simulink model "modelxxx"  (R2023a)
settings: Solver=FixedStepAuto  StartTime=0.0  StopTime=inf  FixedStep=0.001  MaxStep=0.001  RelTol=1e-3
undefined symbols (not defined in the file or in its folder): CR, LF
libraries: instrumentseriallib x2
settings Model: SimulationMode=accelerator  Creator=Adam  LastModifiedBy=Adam
settings SolverCC: AlgebraicLoopSolver=TrustRegion
settings DataIOCC: ExternalInput=ind  SaveOutput=off  SignalLogging=off  DSMLogging=off  SaveTime=off  ReturnWorkspaceOutputs=off  OutputSaveName=out  ReturnWorkspaceOutputsName=sout
settings OptimizationCC: SimCompilerOptimization=on  AccelVerboseBuild=on
settings DebuggingCC: AlgebraicLoopMsg=none  UnconnectedInputMsg=warning  UnconnectedOutputMsg=warning  UnconnectedLineMsg=warning
settings ModelReferenceCC: EnableRefExpFcnMdlSchedulingChecks=on
settings RTWCC: DLArmComputeVersion=19.05

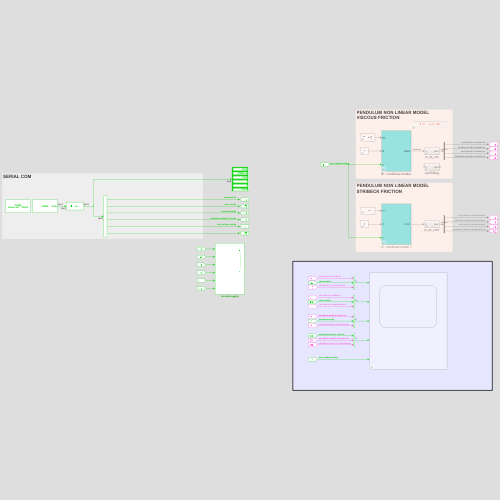
[thumbnail: Simulink's stored preview of the top-level diagram]
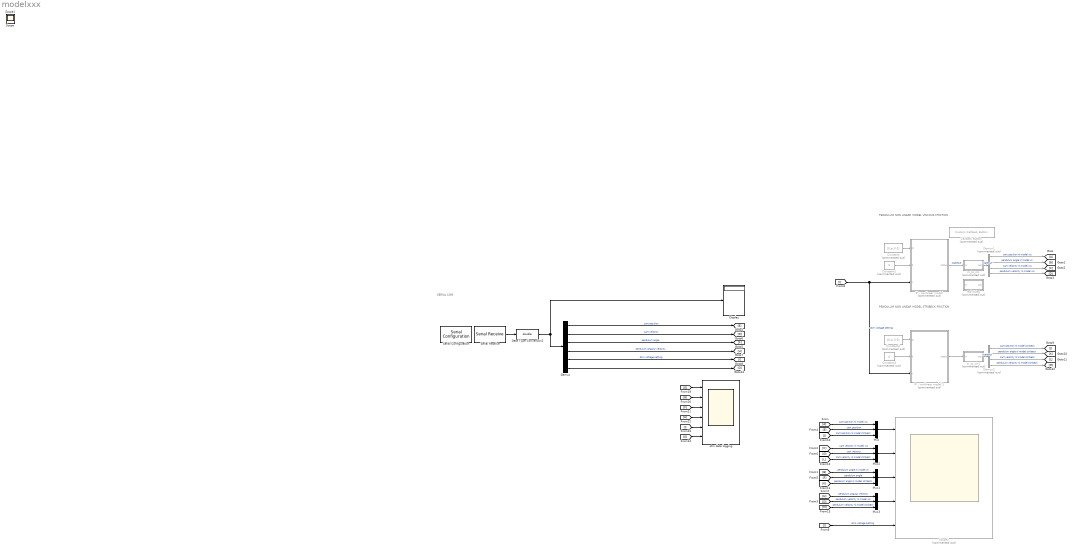
== system modelxxx ==
  note: PENDULUM NON LINEAR MODEL
      | VISCOUS FRICTION
  note: SERIAL COM
  note: PENDULUM NON LINEAR MODEL
      | STRIBECK FRICTION
  Callback Button : CustomCallbackButton  Commented=on  Configuration="{\"components\":[{\"name\":\"BackgroundImageComponent\",\"settings\":{\"image\":{\"size\":[0,0],\"src\":\"default\",\"srcOrientation\":\"Right\"},\"position\":[0,0,1,1]}},{\"name\":\"ButtonStateComponent\",\"settings\":{\"buttonType\":\"momentary\",\"clickFcn\":\"run(\\\"C:\\/adamadam\\/elo\\/ZREPO\\/matlab\\/identyfikacja\\/OK_PARAMETRY_1.m\\\")\",\"onValue\":1,\"position\":[0,0,1,1],\"pressDelay\":\"500\",\"pressFcn\":\"\",\"repeatInterval\":\"0\",\"states\":[{\"horizontalAlignment\":\"center\",\"image\":{\"position\":[0,0,1,1],\"size\":[1,1],\"src\":\"default\",\"srcOrientation\":\"Right\"},\"label\":{\"color\":[1,0,0],\"icon\":{\"size\":[0,0],\"src\":\"default\",\"srcOrientation\":\"Right\"},\"iconPlacement\":\"left\",\"opacity\":1,\"show\":true,\"text\":{\"content\":\"LOAD PARAMS\",\"font\":\"Helvetica\",\"fontSize\":7.199999999999999}},\"labelOffset\":[0,0],\"verticalAlignment\":\"middle\"},{\"horizontalAlignment\":\"center\",\"image\":{\"position\":[0,0,1,1],\"size\":[1,1],\"src\":\"default\",\"srcOrientation\":\"Right\"},\"label\":{\"color\":[0.01176470588,0.01176470588,0.01176470588,1],\"icon\":{\"size\":[0,0],\"src\":\"default\",\"srcOrientation\":\"Right\"},\"iconPlacement\":\"left\",\"opacity\":1,\"show\":true,\"text\":{\"content\":\"LOAD PARAMS\",\"font\":\"Helvetica\",\"fontSize\":7.199999999999999}},\"labelOffset\":[0,0],\"verticalAlignment\":\"middle\"},{\"horizontalAlignment\":\"center\",\"image\":{\"position\":[0,0,1,1],\"size\":[1,1],\"src\":\"default\",\"srcOrientation\":\"Right\"},\"label\":{\"color\":[0.01176470588,0.01176470588,0.01176470588,1],\"icon\":{\"size\":[0,0],\"src\":\"default\",\"srcOrientation\":\"Right\"},\"iconPlacement\":\"left\",\"opacity\":1,\"show\":true,\"text\":{\"content\":\"LOAD PARAMS\",\"font\":\"Helvetica\",\"fontSize\":7.199999999999999}},\"labelOffset\":[0,0],\"verticalAlignment\":\"middle\"},{\"horizontalAlignment\":\"center\",\"image\":{\"position\":[0,0,1,1],\"size\":[1,1],\"src\":\"default\",\"srcOrientation\":\"Right\"},\"label\":{\"color\":[0.01176470588,0.01176470588,0.01176470588,1],\"icon\":{\"size\":[0,0],\"src\":\"default\",\"srcOrientation\":\"Right\"},\"iconPlacement\":\"left\",\"opacity\":1,\"show\":true,\"text\":{\"content\":\"LOAD PARAMS\",\"font\":\"Helvetica\",\"fontSize\":7.199999999999999}},\"labelOffset\":[0,0],\"verticalAlignment\":\"middle\"}]}},{\"name\":\"ForegroundImageComponent\",\"settings\":{\"image\":{\"size\":[0,0],\"src\":\"default\",\"srcOrientation\":\"Right\"},\"isForeground\":1,\"position\":[0,0,1,1]}}],\"settings\":{\"BindingType\":\"standalone\",\"backgroundColor\":[244,244,244,1],\"backgroundOffset\":0.2,\"backgroundOpacity\":1,\"fixedAspectRatio\":\"on\",\"foregroundColor\":[0.01176470588,0.01176470588,0.01176470588,1],\"migratedFromLegacy\":true,\"useBackgroundColor\":true,\"variant\":\"callback\",\"version\":\"R2023a\"},\"type\":\"Button\"}"  CustomBackgroundColor="{\"color\":[0.9568627450980393,0.9568627450980393,0.9568627450980393],\"show\":true}"
  Constant : Constant  Commented=on  Value=[0,pi,0,0]  VectorParams1D=off
  Constant1 : Constant  Commented=on  Value=0
  Constant2 : Constant  Commented=on  Value=[0,pi,0,0]  VectorParams1D=off
  Constant3 : Constant  Commented=on  Value=0
  Data Type Conversion2 : DataTypeConversion  OutDataTypeStr=double  SaturateOnIntegerOverflow=off  RndMeth=Floor
  Demux : Demux  Outputs=6
  Demux1 : Demux  Commented=on
  Demux2 : Demux  Commented=on
  Display : Display
  From : From
  Goto : Goto
  "IP - nonlinear model " : Subsystem  Description=Nonlinear model of inverted pendulum  Commented=on
      mask Display:
      | port_label('output', 1, 'stan');
      | port_label('input', 1, 'IC');
      | port_label('input', 2, 'd');
      | port_label('input', 3, 'v');
  IP - nonlinear model 1 : Subsystem  Description=Nonlinear model of inverted pendulum  Commented=on
      mask Display:
      | port_label('output', 1, 'stan');
      | port_label('input', 1, 'IC');
      | port_label('input', 2, 'd');
      | port_label('input', 3, 'v');
  Mux{,1..3} (4 alike) : Mux  Inputs=3
  Scope2 : Scope  Commented=on  NumInputPorts=5
  Serial Configuration : instrumentseriallib/Serial Configuration  Priority=-200000  PortSel=COM5  Port=COM5  ComPort=COM5  BaudRate=115200  DataBits=8  Parity=none  StopBits=1  ByteOrder=little-endian  FlowControl=none  Timeout=10  SimulateUsing=Interpreted execution  BlockInModel=on  aMode=1
      settings: LibrarySourceBlock=embeddedtargetslib/Host Communication/Serial Configuration
  Serial Receive : instrumentseriallib/Serial Receive  Priority=1  PortSel=COM5  Port=COM5  ComPort=COM5  DataType=single  SaveDataType=uint8  ToggleHeader=off  Header=[]  ToggleTerminator=off  Terminator=CR/LF ('\r\n')  CustomTerminator=[]  InputFormat=Column major  ToggleDataSize=on  DataSize=[6 1]  EnableBlockingMode=on  ActionDataUnavailable=Output last received value  ActionWhenDataUnavailable=Output last received value  CustomValue=0  SampleTime=0.01  SimulateUsing=Interpreted execution  BlockInModel=on  aMode=1
      settings: LibrarySourceBlock=embeddedtargetslib/Host Communication/Serial Receive
  m_to_cm : Subsystem  Commented=on
  m_to_cm1 : Subsystem  Commented=on
  radToDeg : Subsystem  Commented=on
  stm data logging : Scope  NumInputPorts=6
  Scope : Scope
  Scope1 : Scope
  wires:
  Serial Receive/1 -> Data Type Conversion2/1
  Constant/1 -> "IP - nonlinear model "/1(IC)
  Constant1/1 -> "IP - nonlinear model "/2(d)
  "IP - nonlinear model "/1(state) -> m_to_cm/1(in)  "stateout"
  Mux/1 -> Scope2/1
  Mux3/1 -> Scope2/4
  Data Type Conversion2/1 -> Demux/1, Display/1
  Mux2/1 -> Scope2/2
  Mux1/1 -> Scope2/3
  Demux1/1 -> Goto/1  "cart position nl model vis"
  Demux1/2 -> [B]  "pendulum angle nl model vs"
  [B] -> Mux1/1  "pendulum angle nl model vs"
  Demux1/3 -> [C]  "cart velocity nl model vis"
  Demux1/4 -> [D]  "pendulum velocity nl model vis"
  [D] -> Mux3/2  "pendulum velocity nl model vis"
  Demux/1 -> [E]  "cart position"
  [E] -> Mux/2  "cart position"
  [F] -> Mux1/2  "pendulum angle"
  [G] -> Mux2/2  "cart velocity"
  [H] -> Mux3/1  "pendulum angular velocity"
  [I] -> "IP - nonlinear model "/3(v), IP - nonlinear model 1/3(v)  "dcm voltage setting"
  [I] -> Scope2/5  "dcm voltage setting"
  Demux/3 -> [F]  "pendulum angle"
  Demux/2 -> [G]  "cart velocity"
  Demux/4 -> [H]  "pendulum angular velocity"
  Demux/5 -> [I]  "dcm voltage setting"
  From/1 -> Mux/1  "cart position nl model vis"
  [C] -> Mux2/1  "cart velocity nl model vis"
  Constant2/1 -> IP - nonlinear model 1/1(IC)
  Constant3/1 -> IP - nonlinear model 1/2(d)
  IP - nonlinear model 1/1(state) -> m_to_cm1/1(in)
  Demux2/1 -> [J]  "cart position nl model stribeck"
  Demux2/2 -> [K]  "pendulum angle nl model stribeck"
  Demux2/3 -> [L]  "cart velocity nl model stribeck"
  Demux2/4 -> [M]  "pendulum velocity nl model stribeck"
  [J] -> Mux/3  "cart position nl model stribeck"
  m_to_cm/1(out) -> Demux1/1  "stateout"
  m_to_cm1/1(out) -> Demux2/1  "stateout"
  [M] -> Mux3/3  "pendulum velocity nl model stribeck"
  [L] -> Mux2/3  "cart velocity nl model stribeck"
  [K] -> Mux1/3  "pendulum angle nl model stribeck"
  [E] -> stm data logging/1
  [G] -> stm data logging/2
  [F] -> stm data logging/3
  [H] -> stm data logging/4
  [I] -> stm data logging/5
  Demux/6 -> [O]
  [O] -> stm data logging/6

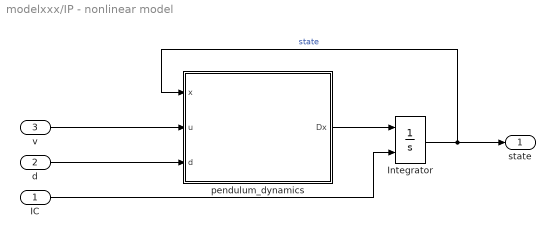
== system modelxxx/IP - nonlinear model  ==
  IC : Inport
  d : Inport  Port=2
  v : Inport  Port=3
  Integrator : Integrator  InitialConditionSource=external
  pendulum_dynamics : MATLAB Function  TreatAsAtomicUnit=on
  state : Outport
  wires:
  Integrator/1 -> state/1, pendulum_dynamics/1(x)  "state"
  v/1 -> pendulum_dynamics/2(u)
  pendulum_dynamics/1(Dx) -> Integrator/1
  IC/1 -> Integrator/2
  d/1 -> pendulum_dynamics/3(d)

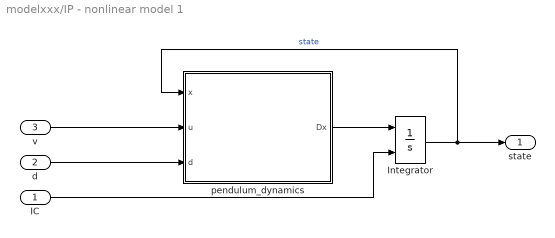
== system modelxxx/IP - nonlinear model 1 ==
  IC : Inport
  d : Inport  Port=2
  v : Inport  Port=3
  Integrator : Integrator  InitialConditionSource=external
  pendulum_dynamics : MATLAB Function  TreatAsAtomicUnit=on
  state : Outport
  wires:
  Integrator/1 -> state/1, pendulum_dynamics/1(x)  "state"
  v/1 -> pendulum_dynamics/2(u)
  pendulum_dynamics/1(Dx) -> Integrator/1
  IC/1 -> Integrator/2
  d/1 -> pendulum_dynamics/3(d)

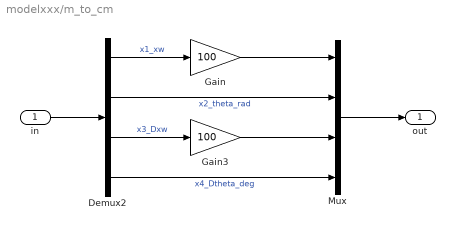
== system modelxxx/m_to_cm ==
  in : Inport
  Demux2 : Demux
  Gain : Gain  Gain=100
  Gain3 : Gain  Gain=100
  Mux : Mux
  out : Outport
  wires:
  Demux2/1 -> Gain/1  "x1_xw"
  Demux2/4 -> Mux/4  "x4_Dtheta_deg"
  Demux2/2 -> Mux/2  "x2_theta_rad"
  in/1 -> Demux2/1
  Demux2/3 -> Gain3/1  "x3_Dxw"
  Mux/1 -> out/1
  Gain/1 -> Mux/1
  Gain3/1 -> Mux/3

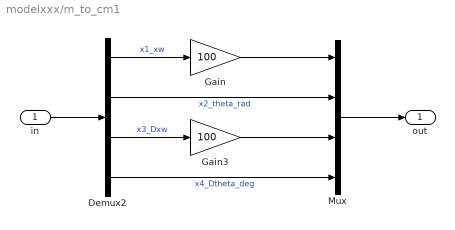
== system modelxxx/m_to_cm1 ==
  in : Inport
  Demux2 : Demux
  Gain : Gain  Gain=100
  Gain3 : Gain  Gain=100
  Mux : Mux
  out : Outport
  wires:
  Demux2/1 -> Gain/1  "x1_xw"
  Demux2/4 -> Mux/4  "x4_Dtheta_deg"
  Demux2/2 -> Mux/2  "x2_theta_rad"
  in/1 -> Demux2/1
  Demux2/3 -> Gain3/1  "x3_Dxw"
  Mux/1 -> out/1
  Gain/1 -> Mux/1
  Gain3/1 -> Mux/3

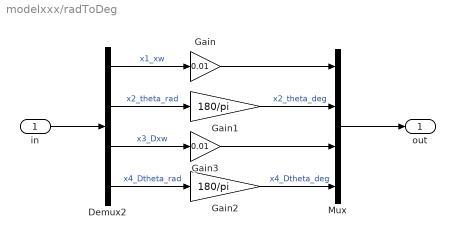
== system modelxxx/radToDeg ==
  in : Inport
  Demux2 : Demux
  Gain : Gain  Gain=0.01
  Gain1 : Gain  Gain=180/pi
  Gain2 : Gain  Gain=180/pi
  Gain3 : Gain  Gain=0.01
  Mux : Mux
  out : Outport
  wires:
  Demux2/1 -> Gain/1  "x1_xw"
  Gain1/1 -> Mux/2  "x2_theta_deg"
  Gain2/1 -> Mux/4  "x4_Dtheta_deg"
  Demux2/2 -> Gain1/1  "x2_theta_rad"
  in/1 -> Demux2/1
  Demux2/3 -> Gain3/1  "x3_Dxw"
  Demux2/4 -> Gain2/1  "x4_Dtheta_rad"
  Mux/1 -> out/1
  Gain/1 -> Mux/1
  Gain3/1 -> Mux/3

== matlab function modelxxx/IP - nonlinear model 1/pendulum_dynamics ==
  data: x input; u input; d input; Dx output; params_stribeck parameter
function Dx = dynamika_wahadla(x, u, d, params_stribeck)
% x : stan
% u : input - napięcie
%
% params scope: "parameters"
%

% State, function input: x = [x Dx theta Dtheta]'
x1 = x(1);
x2 = x(2);
x3 = x(3);
x4 = x(4);
 
params_stribeck = num2cell(params_stribeck);
[M, mc, mp, Lp, Lc, g, b_stribeck, gamma, mr, Mt, L, Jcm, Jt, alpha, beta, miu_c, miu_s, vs, i_, delta] = params_stribeck{:};

% Equations for pendulum dynamics
Ff = (miu_c + (miu_s-miu_c)*exp(-(x3/vs)^i_)) * Mt*g*tanh(delta*x3) + b_stribeck*x3;
Fi = alpha*u - beta*x3;
A = d*cos(x2) - Ff + L*mr*x4^2*sin(x2) + Fi;
B = d*Lc + L*g*mr*sin(x2) - gamma*x4;
DEN = Jt*Mt - (L*mr*cos(x2))^2;

ddt_x1 = x3;
ddt_x2 = x4;
ddt_x3 = (Jt*A - L*mr*cos(x2)*B) / DEN;
ddt_x4 = (Mt*B - L*mr*cos(x2)*A) / DEN;

% output
Dx = [ddt_x1 ddt_x2 ddt_x3 ddt_x4]';

end

== matlab function modelxxx/IP - nonlinear model /pendulum_dynamics ==
  data: x input; u input; d input; Dx output; params_lepkie parameter
function Dx = pendulum_dynamics(x, u, d, params_lepkie)
% x : state
% u : input - napięcie
%
% params scope: "parameters"
%

% State, function input: x = [x Dx theta Dtheta]'
x1 = x(1);
x2 = x(2); 
x3 = x(3);
x4 = x(4);

% if (x1 >= 0.47)
%    x1 = 0.47;
%    x2 = 0;
% elseif (x1 <= 0)
%    x1 = 0;
%    x2 = 0;
% end

params_lepkie = num2cell(params_lepkie);
[M, mc, mp, Lp, Lc, g, b, gamma, mr, Mt, L, Jcm, Jt, alpha, beta] = params_lepkie{:};

% Equations for pendulum dynamics
Ff = b*x3;
Fi = alpha*u - beta*x3;
A = d*cos(x2) - Ff + L*mr*x4^2*sin(x2) + Fi;
B = d*Lc + L*g*mr*sin(x2) - gamma*x4;
DEN = Jt*Mt - (L*mr*cos(x2))^2;

ddt_x1 = x3;
ddt_x2 = x4;
ddt_x3 = (Jt*A - L*mr*cos(x2)*B) / DEN;
ddt_x4 = (Mt*B - L*mr*cos(x2)*A) / DEN;

% output (column vector)
Dx = [ddt_x1 ddt_x2 ddt_x3 ddt_x4]';

end
